simulink model "adc_to_xaui_v2_ddc"  (Simulink 6.2)
settings: Solver=ode45  StartTime=0.0  StopTime=100  RelTol=1e-3
undefined symbols (not defined in the file): BitWidth, iBOB
libraries: xbsIndex_r3 x168, casper_library x18, xps_library x5
(part 1 of 3)
settings Model: LastModifiedBy=siemion
settings DebuggingCC: SolverPrmCheckMsg=warning

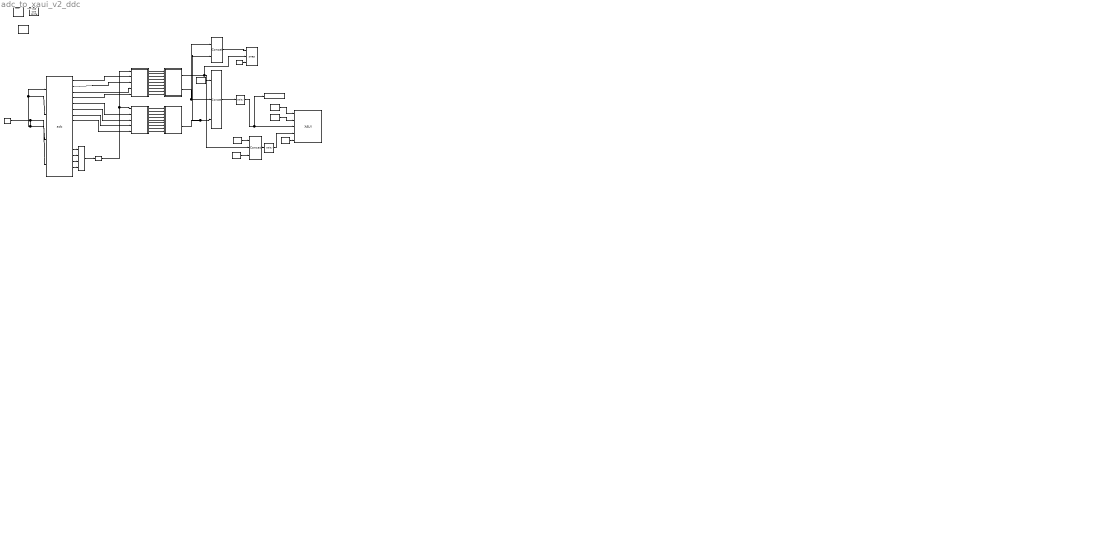
== system adc_to_xaui_v2_ddc ==
  note: left
  note: ADC-to-XAUI
      | Author: Peter McMahon
      | Version: 1.0
      | February 2008
  note: Beamformer Output:
      |
      | outofband[0]: 100PPS
      | outofband[1]: 1PPS
      | outofband[2-7]: unused
      |
      | data[0-7]: Pol 1 I
      | data[8-15]: Pol 1 Q
      | data[16-23]: Pol 2 I
      | data[24-31]: Pol 2 Q
      | data[31-63]: unused
  note: Used as a test device to emulate ATA beamformer.
      |
      | Digitizes data from 2x I/Q streams, and outputs them over XAUI.
  note: Pol 1
  note: Delay:
      | 1.) You always need at least one delay.
      | 2.) We want a delay of 5 to see if we can measure the
      | delay in the 1PPS in the ata_xaui design.
  " System Generator" : xbsIndex_r3/ System Generator  Tag=genX  xilinxfamily=Virtex2P  part=xc2vp50  speed=-7  package=ff1152  synthesis_tool=XST  directory=./adc_to_xaui_v2_ddc/sysgen  testbench=off  simulink_period=1  sysclk_period=8  incr_netlist=off  trim_vbits=Everywhere in SubSystem  dbl_ovrd=According to Block Masks  core_generation=According to Block Masks  run_coregen=off  deprecated_control=off  eval_field=0
      settings: AttributesFormatString=System\nGenerator
  Delay : xbsIndex_r3/Delay  latency=5  reg_retiming=off  explicit_period=off  period=1  en=off  accept_only_valid=off  init_zero=on  dbl_ovrd=off  show_param=off
      settings: xl_area=[0, 0, 0, 0, 0, 0, 0]
  Delay1 : xbsIndex_r3/Delay  latency=5  reg_retiming=off  explicit_period=off  period=1  en=off  accept_only_valid=off  init_zero=on  dbl_ovrd=off  show_param=off
      settings: xl_area=[0, 0, 0, 0, 0, 0, 0]
  XAUI : xps_library/XAUI  Tag=xps:xaui  demux=1  port=iBOB:1  show_param=on  pre_emph=2  swing=800
  XSG core config : xps_library/XSG core config  Tag=xps:xsg  hw_sys=iBOB  ibob_linux=off  clk_src=adc0_clk  gpio_clk_io_group=iBOB:sma  gpio_clk_bit_index=0  clk_rate=125  sample_period=1  synthesis_tool=XST  mpc_type=powerpc405
  adc : xps_library/adc  Tag=xps:adc  adc_brd=iBOB:adc0  adc_clk_rate=500  adc_interleave=off  sample_period=1
  cns0_2 : xbsIndex_r3/Constant  const=0  equ=P=C  arith_type=Boolean  n_bits=1  bin_pt=0  opselect=C  inp2=PCIN>>17  opr=+  inp1=P  carry=CIN  iostate=0  explicit_period=on  period=1  dbl_ovrd=off
  cns_xaui_data_32bits : xbsIndex_r3/Constant  const=0  equ=P=C  arith_type=Unsigned  n_bits=32  bin_pt=0  opselect=C  inp2=PCIN>>17  opr=+  inp1=P  carry=CIN  iostate=0  explicit_period=on  period=1  dbl_ovrd=off
  cns_xaui_outofband_1bit : xbsIndex_r3/Constant  const=0  equ=P=C  arith_type=Unsigned  n_bits=1  bin_pt=0  opselect=C  inp2=PCIN>>17  opr=+  inp1=P  carry=CIN  iostate=0  explicit_period=on  period=1  dbl_ovrd=off
  cns_xaui_outofband_6bits : xbsIndex_r3/Constant  const=0  equ=P=C  arith_type=Unsigned  n_bits=6  bin_pt=0  opselect=C  inp2=PCIN>>17  opr=+  inp1=P  carry=CIN  iostate=0  explicit_period=on  period=1  dbl_ovrd=off
  cns_xaui_rx_get : xbsIndex_r3/Constant  const=1  equ=P=C  arith_type=Boolean  n_bits=1  bin_pt=0  opselect=C  inp2=PCIN>>17  opr=+  inp1=P  carry=CIN  iostate=0  explicit_period=on  period=1  dbl_ovrd=off
  cns_xaui_rx_reset : xbsIndex_r3/Constant  const=0  equ=P=C  arith_type=Boolean  n_bits=1  bin_pt=0  opselect=C  inp2=PCIN>>17  opr=+  inp1=P  carry=CIN  iostate=0  explicit_period=on  period=1  dbl_ovrd=off
  cns_xaui_tx_valid : xbsIndex_r3/Constant  const=1  equ=P=C  arith_type=Boolean  n_bits=8  bin_pt=0  opselect=C  inp2=PCIN>>17  opr=+  inp1=P  carry=CIN  iostate=0  explicit_period=on  period=1  dbl_ovrd=off
  concat_data : xbsIndex_r3/Concat  num_inputs=3  explicit_period=off  period=1  dbl_ovrd=off
  concat_data1 : xbsIndex_r3/Concat  num_inputs=2  explicit_period=off  period=1  dbl_ovrd=off
  concat_outofband : xbsIndex_r3/Concat  num_inputs=3  explicit_period=off  period=1  dbl_ovrd=off
  dec_fir : Subsystem  AncestorBlock=casper_library/Downconverter/dec_fir  mask(dec_fir){n_inputs=4, coeff=.9 * [-0.0161   -0.0428   -0.0504   -0.0249    0.0354    0.1170    0.1948    0.2422    0.2422    0.1948    0.1170  0.0354   -0.0249   -0.0504   -0.0428   -0.0161], n_bits=8, quantization=Round  (unbiased: Even Values), add_latency=2, mult_latency=2}
      mask prompts: n_inputs "Number of Parallel Streams"; coeff "Coefficients"; n_bits "Bit Width Out"; quantization "Quantization Behavior"; add_latency "Add Latency"; mult_latency "Mult Latency"
      mask help: FIR filter which can handle multiple time samples in parallel and decimates down to 1 time sample. If coefficients are symmetric, will automatically fold before multiplying.
      mask init:
      | dec_fir_init(gcb, ...
      |     'n_inputs', n_inputs, ...
      |     'coeff', coeff, ...
      |     'n_bits', n_bits, ...
      |     'quantization', quantization, ...
      |     'add_latency', add_latency, ...
      |     'mult_latency', mult_latency);
      settings: AttributesFormatString=|
      | 16 taps
      | 8_7 r/i
      mask Help:
      | <h1>Description</h1>
      | 
      | FIR filter which can handle multiple time samples in parallel and decimates down to 1 time sample.  If coefficients are symmetric, will automatically fold before multiplying.
      | 
      | <h2>Mask Parameters</h2>
      | 
      | <b>Number of Parallel Streams</b> (n_inputs): The number of time samples which arrive in parallel.<br><br>
      | 
      | <b>Coefficients</b> (coeff): The FIR coefficients.  If this vector is symmetric, the FIR will automatically fold before multiplying.<br><br>
      | 
      | <b>Bit Width Out</b> (n_bits): The number of bits in each real/imag sample of the complex number that is output.<br><br>
      | 
      | <b>Quantization Behavior</b> (quantization): The quantization behavior used in converting to the output bit width.<br><br>
      | 
      | 
      | <b>Add Latency</b> (add_latency) = The latency of adders/converters.<br><br>
      | 
      | <b>Mult Latency</b> (mult_latency) = The latency of multipliers.<br><br>
      mask StyleString: edit,edit,edit,popup(Truncate|Round  (unbiased: +/- Inf)|Round  (unbiased: Even Values)),edit,edit
  dec_fir1 : Subsystem  AncestorBlock=casper_library/Downconverter/dec_fir  mask(dec_fir){n_inputs=4, coeff=.9 * [-0.0161   -0.0428   -0.0504   -0.0249    0.0354    0.1170    0.1948    0.2422    0.2422    0.1948    0.1170  0.0354   -0.0249   -0.0504   -0.0428   -0.0161], n_bits=8, quantization=Round  (unbiased: Even Values), add_latency=2, mult_latency=2}
      mask prompts: n_inputs "Number of Parallel Streams"; coeff "Coefficients"; n_bits "Bit Width Out"; quantization "Quantization Behavior"; add_latency "Add Latency"; mult_latency "Mult Latency"
      mask help: FIR filter which can handle multiple time samples in parallel and decimates down to 1 time sample. If coefficients are symmetric, will automatically fold before multiplying.
      mask init: same as adc_to_xaui_v2_ddc/dec_fir
      settings: AttributesFormatString=|
      | 16 taps
      | 8_7 r/i
      mask Help:
      | <h1>Description</h1>
      | 
      | FIR filter which can handle multiple time samples in parallel and decimates down to 1 time sample.  If coefficients are symmetric, will automatically fold before multiplying.
      | 
      | <h2>Mask Parameters</h2>
      | 
      | <b>Number of Parallel Streams</b> (n_inputs): The number of time samples which arrive in parallel.<br><br>
      | 
      | <b>Coefficients</b> (coeff): The FIR coefficients.  If this vector is symmetric, the FIR will automatically fold before multiplying.<br><br>
      | 
      | <b>Bit Width Out</b> (n_bits): The number of bits in each real/imag sample of the complex number that is output.<br><br>
      | 
      | <b>Quantization Behavior</b> (quantization): The quantization behavior used in converting to the output bit width.<br><br>
      | 
      | 
      | <b>Add Latency</b> (add_latency) = The latency of adders/converters.<br><br>
      | 
      | <b>Mult Latency</b> (mult_latency) = The latency of multipliers.<br><br>
      mask StyleString: edit,edit,edit,popup(Truncate|Round  (unbiased: +/- Inf)|Round  (unbiased: Even Values)),edit,edit
  ibob_lwip : xps_library/ibob_lwip
  mixer : Subsystem  AncestorBlock=casper_library/Downconverter/mixer  mask(mixer){freq_div=4, freq=1, nstreams=4, n_bits=8, bram_latency=2, mult_latency=3}
      mask prompts: freq_div "Frequency Divisions (M)"; freq "Mixing Frequency (? / M*2pi)"; nstreams "Number of Parallel Streams"; n_bits "Bit Width"; bram_latency "BRAM Latency"; mult_latency "Mult Latency"
      mask help: Digitally mixes an input signal (which can be several samples in parallel) with an LO of the indicated frequency (which is some fraction of the native FPGA clock rate).
      mask init:
      | mixer_init(gcb, ...
      |     'freq_div', freq_div, ...
      |     'freq', freq, ...
      |     'nstreams', nstreams, ...
      |     'n_bits', n_bits, ...
      |     'bram_latency', bram_latency, ...
      |     'mult_latency', mult_latency);
      settings: AttributesFormatString=lo at -1/4
      mask Help:
      | <h1>Description</h1>
      | 
      | Digitally mixes an input signal (which can be several samples in parallel) with an LO of the indicated frequency (which is some fraction of the native FPGA clock rate).
      | 
      | <h2>Mask Parameters</h2>
      | 
      | <b>Frequency Divisions</b> (freq_div):  The (power of 2) denominator of the mixing frequency. <br><br>
      | 
      | <b>Mixing Frequency</b> (freq) = The numerator of the mixing frequency.<br><br>
      | 
      | <b>Number of Parallel Streams</b> (nstreams) = The number of samples which arrive in parallel.<br><br>
      | 
      | <b>Bit Width</b> (n_bits) = The bitwidth of LO samples.<br><br>
      | 
      | <b>BRAM Latency</b> (bram_latency) = The latency of sine/cos lookup table.<br><br>
      | 
      | <b>MULT Latency</b> (mult_latency) = The latency of mixing multipliers.<br><br>
      | 
      | <h2> Usage </h2>
      | M = Frequency Divisions<br>
      | F = Mixing Frequency<br>
      | M and F must both be integers, and M must be a power of 2. The ratio F/M should equal the ratio f/r where r is the data rate of the sampled signal. For example, an F/M of 3/16 would downmix an 800Msps signal with an LO of 150MHz.
  mixer1 : Subsystem  AncestorBlock=casper_library/Downconverter/mixer  mask(mixer){freq_div=4, freq=1, nstreams=4, n_bits=8, bram_latency=2, mult_latency=3}
      mask prompts: freq_div "Frequency Divisions (M)"; freq "Mixing Frequency (? / M*2pi)"; nstreams "Number of Parallel Streams"; n_bits "Bit Width"; bram_latency "BRAM Latency"; mult_latency "Mult Latency"
      mask help: Digitally mixes an input signal (which can be several samples in parallel) with an LO of the indicated frequency (which is some fraction of the native FPGA clock rate).
      mask init: same as adc_to_xaui_v2_ddc/mixer
      settings: AttributesFormatString=lo at -1/4
      mask Help:
      | <h1>Description</h1>
      | 
      | Digitally mixes an input signal (which can be several samples in parallel) with an LO of the indicated frequency (which is some fraction of the native FPGA clock rate).
      | 
      | <h2>Mask Parameters</h2>
      | 
      | <b>Frequency Divisions</b> (freq_div):  The (power of 2) denominator of the mixing frequency. <br><br>
      | 
      | <b>Mixing Frequency</b> (freq) = The numerator of the mixing frequency.<br><br>
      | 
      | <b>Number of Parallel Streams</b> (nstreams) = The number of samples which arrive in parallel.<br><br>
      | 
      | <b>Bit Width</b> (n_bits) = The bitwidth of LO samples.<br><br>
      | 
      | <b>BRAM Latency</b> (bram_latency) = The latency of sine/cos lookup table.<br><br>
      | 
      | <b>MULT Latency</b> (mult_latency) = The latency of mixing multipliers.<br><br>
      | 
      | <h2> Usage </h2>
      | M = Frequency Divisions<br>
      | F = Mixing Frequency<br>
      | M and F must both be integers, and M must be a power of 2. The ratio F/M should equal the ratio f/r where r is the data rate of the sampled signal. For example, an F/M of 3/16 would downmix an 800Msps signal with an LO of 150MHz.
  posedge : casper_library/Misc/posedge  Tag=Rising Edge Detector
  reg_xauiscope1 : xps_library/software register  Tag=xps:sw_reg  io_dir=To Processor  arith_type=Unsigned  bitwidth=32  bin_pt=0  sample_period=1  gw_name=adc_to_xaui_v2_ddc_reg_xauiscope1_user_data_in
  sim_zero : Constant  Value=0
  snap_ddc : casper_library/Scopes/snap  nsamples=11
  sync_or : xbsIndex_r3/Logical  logical_function=OR  inputs=4  precision=Full  arith_type=Unsigned  n_bits=8  bin_pt=2  align_bp=on  latency=1  explicit_period=off  period=1  en=off  dbl_ovrd=off  show_param=off
      settings: xl_area=[0, 0, 0, 0, 0, 0, 0]
  wires:
  sim_zero/1 -> adc/4, adc/3, adc/2, adc/1
  adc/13 -> sync_or/1
  adc/14 -> sync_or/2
  adc/15 -> sync_or/3
  adc/16 -> sync_or/4
  sync_or/1 -> posedge/1
  cns_xaui_rx_get/1 -> XAUI/1
  cns_xaui_rx_reset/1 -> XAUI/2
  concat_outofband/1 -> Delay1/1
  cns_xaui_tx_valid/1 -> XAUI/5
  cns_xaui_data_32bits/1 -> concat_data/1
  cns_xaui_outofband_6bits/1 -> concat_outofband/1
  cns_xaui_outofband_1bit/1 -> concat_outofband/3
  concat_data/1 -> Delay/1
  Delay/1 -> XAUI/3, reg_xauiscope1/1
  Delay1/1 -> XAUI/4
  mixer/1(sync_out) -> dec_fir/1(sync_in)
  mixer/2(real1) -> dec_fir/2(real1)
  mixer/3(imag1) -> dec_fir/3(imag1)
  mixer/4(real2) -> dec_fir/4(real2)
  mixer/5(imag2) -> dec_fir/5(imag2)
  mixer/6(real3) -> dec_fir/6(real3)
  mixer/7(imag3) -> dec_fir/7(imag3)
  mixer/8(real4) -> dec_fir/8(real4)
  mixer/9(imag4) -> dec_fir/9(imag4)
  mixer1/1(sync_out) -> dec_fir1/1(sync_in)
  mixer1/2(real1) -> dec_fir1/2(real1)
  mixer1/3(imag1) -> dec_fir1/3(imag1)
  mixer1/4(real2) -> dec_fir1/4(real2)
  mixer1/5(imag2) -> dec_fir1/5(imag2)
  mixer1/6(real3) -> dec_fir1/6(real3)
  mixer1/7(imag3) -> dec_fir1/7(imag3)
  mixer1/8(real4) -> dec_fir1/8(real4)
  mixer1/9(imag4) -> dec_fir1/9(imag4)
  adc/1 -> mixer/2(din1)
  adc/2 -> mixer/3(din2)
  adc/3 -> mixer/4(din3)
  adc/4 -> mixer/5(din4)
  adc/5 -> mixer1/2(din1)
  adc/6 -> mixer1/3(din2)
  adc/7 -> mixer1/4(din3)
  adc/8 -> mixer1/5(din4)
  dec_fir/2(dout) -> concat_data/2, concat_data1/1
  dec_fir1/2(dout) -> concat_data/3, concat_data1/2
  posedge/1 -> mixer/1(sync), mixer1/1(sync)
  dec_fir/1(sync_out) -> concat_outofband/2, snap_ddc/2
  cns0_2/1 -> snap_ddc/3
  concat_data1/1 -> snap_ddc/1

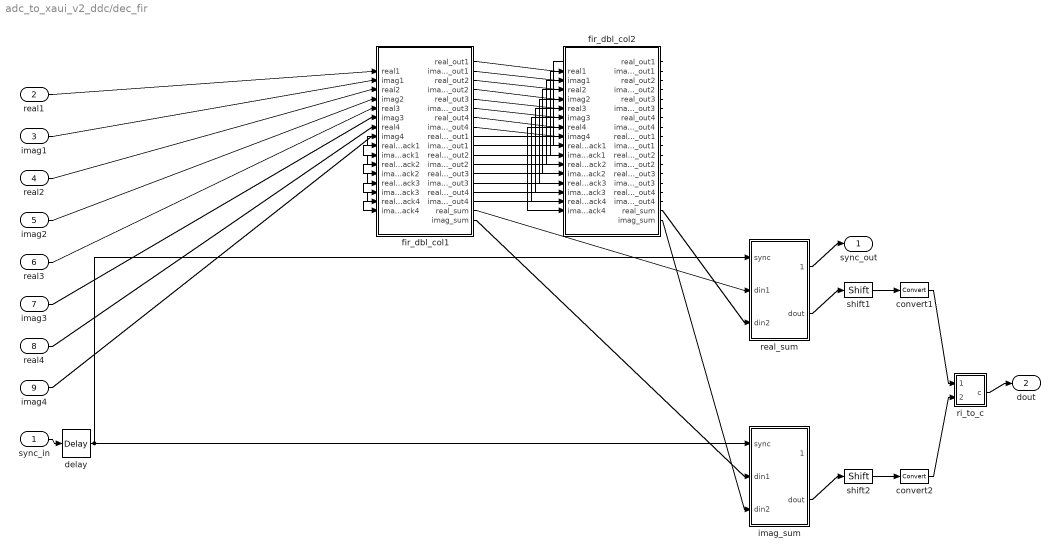
== system adc_to_xaui_v2_ddc/dec_fir ==
  sync_in : Inport  Port=1  LatchInput=off
  real1 : Inport  Port=2  LatchInput=off
  imag1 : Inport  Port=3  LatchInput=off
  real2 : Inport  Port=4  LatchInput=off
  imag2 : Inport  Port=5  LatchInput=off
  real3 : Inport  Port=6  LatchInput=off
  imag3 : Inport  Port=7  LatchInput=off
  real4 : Inport  Port=8  LatchInput=off
  imag4 : Inport  Port=9  LatchInput=off
  convert1 : xbsIndex_r3/Convert  arith_type="Signed  (2's comp)"  n_bits=8  bin_pt=7  quantization="Round  (unbiased: Even Values)"  overflow=Saturate  latency=2  explicit_period=on  period=1  dbl_ovrd=off  show_param=on  inserted_by_tool=off  pipeline=on
      settings: xl_area=[0, 0, 0, 0, 0, 0, 0]
  convert2 : xbsIndex_r3/Convert  arith_type="Signed  (2's comp)"  n_bits=8  bin_pt=7  quantization="Round  (unbiased: Even Values)"  overflow=Saturate  latency=2  explicit_period=on  period=1  dbl_ovrd=off  show_param=on  inserted_by_tool=off  pipeline=on
      settings: xl_area=[0, 0, 0, 0, 0, 0, 0]
  delay : xbsIndex_r3/Delay  latency=12  reg_retiming=off  explicit_period=off  period=1  en=off  accept_only_valid=off  init_zero=on  dbl_ovrd=off  show_param=off
      settings: xl_area=[0, 0, 0, 0, 0, 0, 0]
  fir_dbl_col1 : Subsystem  AncestorBlock=casper_library/Downconverter/fir_dbl_col  mask(fir_dbl_col){n_inputs=4, coeff=[-0.02241 -0.04536 -0.03852 -0.01449], add_latency=2, mult_latency=2}
      mask prompts: n_inputs "Inputs"; coeff "Coefficients"; add_latency "Add latency"; mult_latency "Mult Latency"
      mask init:
      | fir_dbl_col_init(gcb, ...
      |     'n_inputs', n_inputs, ...
      |     'coeff', coeff, ...
      |     'mult_latency', mult_latency, ...
      |     'add_latency', add_latency);
  fir_dbl_col2 : Subsystem  AncestorBlock=casper_library/Downconverter/fir_dbl_col  mask(fir_dbl_col){n_inputs=4, coeff=[0.21798 0.17532 0.1053 0.03186], add_latency=2, mult_latency=2}
      mask prompts: n_inputs "Inputs"; coeff "Coefficients"; add_latency "Add latency"; mult_latency "Mult Latency"
      mask init:
      | fir_dbl_col_init(gcb, ...
      |     'n_inputs', n_inputs, ...
      |     'coeff', coeff, ...
      |     'mult_latency', mult_latency, ...
      |     'add_latency', add_latency);
  imag_sum : Subsystem  AncestorBlock=casper_library/Misc/adder_tree  mask(adder_tree){n_inputs=2, latency=2}
      mask prompts: n_inputs "Number of Inputs"; latency "Add Latency"
      mask help: Sums all inputs using a tree of adds and delays.
      mask init:
      | adder_tree_init(gcb, ...
      |     'n_inputs', n_inputs, ...
      |     'latency', latency);
      settings: AttributesFormatString=latency 2
      mask Help: eval('xlWeb([getenv(''MLIB_ROOT''), ''\doc\html\sp_adder_tree\sp_adder_tree.html''])')
  real_sum : Subsystem  AncestorBlock=casper_library/Misc/adder_tree  mask(adder_tree){n_inputs=2, latency=2}
      mask prompts: n_inputs "Number of Inputs"; latency "Add Latency"
      mask help: Sums all inputs using a tree of adds and delays.
      mask init:
      | adder_tree_init(gcb, ...
      |     'n_inputs', n_inputs, ...
      |     'latency', latency);
      settings: AttributesFormatString=latency 2
      mask Help: eval('xlWeb([getenv(''MLIB_ROOT''), ''\doc\html\sp_adder_tree\sp_adder_tree.html''])')
  ri_to_c : Subsystem
  shift1 : xbsIndex_r3/Shift  shift_dir=Left  shift_bits=1  precision=Full  arith_type="Signed  (2's comp)"  n_bits=8  bin_pt=2  quantization=Truncate  overflow=Wrap  latency=0  explicit_period=off  period=1  en=off  dbl_ovrd=off  show_param=off
      settings: xl_area=[0, 0, 0, 0, 0, 0, 0]
  shift2 : xbsIndex_r3/Shift  shift_dir=Left  shift_bits=1  precision=Full  arith_type="Signed  (2's comp)"  n_bits=8  bin_pt=2  quantization=Truncate  overflow=Wrap  latency=0  explicit_period=off  period=1  en=off  dbl_ovrd=off  show_param=off
      settings: xl_area=[0, 0, 0, 0, 0, 0, 0]
  sync_out : Outport
  dout : Outport  Port=2
  wires:
  real1/1 -> fir_dbl_col1/1(real1)
  imag1/1 -> fir_dbl_col1/2(imag1)
  real2/1 -> fir_dbl_col1/3(real2)
  imag2/1 -> fir_dbl_col1/4(imag2)
  real3/1 -> fir_dbl_col1/5(real3)
  imag3/1 -> fir_dbl_col1/6(imag3)
  real4/1 -> fir_dbl_col1/7(real4)
  imag4/1 -> fir_dbl_col1/8(imag4)
  fir_dbl_col1/17(real_sum) -> real_sum/2(din1)
  fir_dbl_col1/18(imag_sum) -> imag_sum/2(din1)
  fir_dbl_col1/1(real_out1) -> fir_dbl_col2/1(real1)
  fir_dbl_col1/2(imag_out1) -> fir_dbl_col2/2(imag1)
  fir_dbl_col1/3(real_out2) -> fir_dbl_col2/3(real2)
  fir_dbl_col1/4(imag_out2) -> fir_dbl_col2/4(imag2)
  fir_dbl_col1/5(real_out3) -> fir_dbl_col2/5(real3)
  fir_dbl_col1/6(imag_out3) -> fir_dbl_col2/6(imag3)
  fir_dbl_col1/7(real_out4) -> fir_dbl_col2/7(real4)
  fir_dbl_col1/8(imag_out4) -> fir_dbl_col2/8(imag4)
  fir_dbl_col2/17(real_sum) -> real_sum/3(din2)
  fir_dbl_col2/18(imag_sum) -> imag_sum/3(din2)
  real_sum/2(dout) -> shift1/1
  imag_sum/2(dout) -> shift2/1
  shift1/1 -> convert1/1
  shift2/1 -> convert2/1
  convert1/1 -> ri_to_c/1(re)
  convert2/1 -> ri_to_c/2(im)
  ri_to_c/1(c) -> dout/1
  sync_in/1 -> delay/1
  delay/1 -> real_sum/1(sync), imag_sum/1(sync)
  real_sum/1(sync_out) -> sync_out/1
  fir_dbl_col2/9(real_back_out1) -> fir_dbl_col1/9(real_back1)
  fir_dbl_col2/10(imag_back_out1) -> fir_dbl_col1/10(imag_back1)
  fir_dbl_col2/11(real_back_out2) -> fir_dbl_col1/11(real_back2)
  fir_dbl_col2/12(imag_back_out2) -> fir_dbl_col1/12(imag_back2)
  fir_dbl_col2/13(real_back_out3) -> fir_dbl_col1/13(real_back3)
  fir_dbl_col2/14(imag_back_out3) -> fir_dbl_col1/14(imag_back3)
  fir_dbl_col2/15(real_back_out4) -> fir_dbl_col1/15(real_back4)
  fir_dbl_col2/16(imag_back_out4) -> fir_dbl_col1/16(imag_back4)
  fir_dbl_col2/1(real_out1) -> fir_dbl_col2/9(real_back1)
  fir_dbl_col2/2(imag_out1) -> fir_dbl_col2/10(imag_back1)
  fir_dbl_col2/3(real_out2) -> fir_dbl_col2/11(real_back2)
  fir_dbl_col2/4(imag_out2) -> fir_dbl_col2/12(imag_back2)
  fir_dbl_col2/5(real_out3) -> fir_dbl_col2/13(real_back3)
  fir_dbl_col2/6(imag_out3) -> fir_dbl_col2/14(imag_back3)
  fir_dbl_col2/7(real_out4) -> fir_dbl_col2/15(real_back4)
  fir_dbl_col2/8(imag_out4) -> fir_dbl_col2/16(imag_back4)

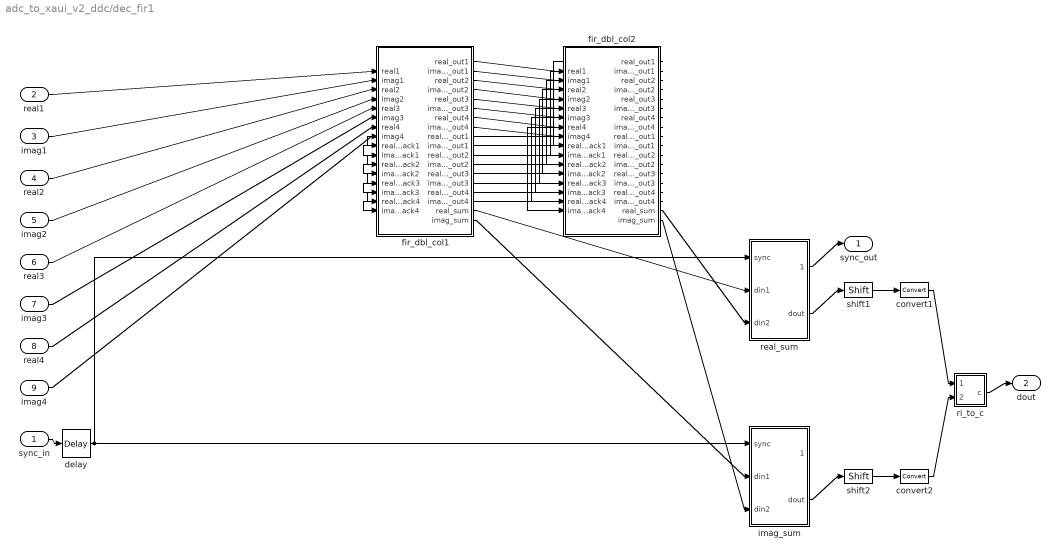
== system adc_to_xaui_v2_ddc/dec_fir1 ==
  sync_in : Inport  Port=1  LatchInput=off
  real1 : Inport  Port=2  LatchInput=off
  imag1 : Inport  Port=3  LatchInput=off
  real2 : Inport  Port=4  LatchInput=off
  imag2 : Inport  Port=5  LatchInput=off
  real3 : Inport  Port=6  LatchInput=off
  imag3 : Inport  Port=7  LatchInput=off
  real4 : Inport  Port=8  LatchInput=off
  imag4 : Inport  Port=9  LatchInput=off
  convert1 : xbsIndex_r3/Convert  arith_type="Signed  (2's comp)"  n_bits=8  bin_pt=7  quantization="Round  (unbiased: Even Values)"  overflow=Saturate  latency=2  explicit_period=on  period=1  dbl_ovrd=off  show_param=on  inserted_by_tool=off  pipeline=on
      settings: xl_area=[0, 0, 0, 0, 0, 0, 0]
  convert2 : xbsIndex_r3/Convert  arith_type="Signed  (2's comp)"  n_bits=8  bin_pt=7  quantization="Round  (unbiased: Even Values)"  overflow=Saturate  latency=2  explicit_period=on  period=1  dbl_ovrd=off  show_param=on  inserted_by_tool=off  pipeline=on
      settings: xl_area=[0, 0, 0, 0, 0, 0, 0]
  delay : xbsIndex_r3/Delay  latency=12  reg_retiming=off  explicit_period=off  period=1  en=off  accept_only_valid=off  init_zero=on  dbl_ovrd=off  show_param=off
      settings: xl_area=[0, 0, 0, 0, 0, 0, 0]
  fir_dbl_col1 : Subsystem  AncestorBlock=casper_library/Downconverter/fir_dbl_col  mask(fir_dbl_col){n_inputs=4, coeff=[-0.02241 -0.04536 -0.03852 -0.01449], add_latency=2, mult_latency=2}
      mask prompts: n_inputs "Inputs"; coeff "Coefficients"; add_latency "Add latency"; mult_latency "Mult Latency"
      mask init:
      | fir_dbl_col_init(gcb, ...
      |     'n_inputs', n_inputs, ...
      |     'coeff', coeff, ...
      |     'mult_latency', mult_latency, ...
      |     'add_latency', add_latency);
  fir_dbl_col2 : Subsystem  AncestorBlock=casper_library/Downconverter/fir_dbl_col  mask(fir_dbl_col){n_inputs=4, coeff=[0.21798 0.17532 0.1053 0.03186], add_latency=2, mult_latency=2}
      mask prompts: n_inputs "Inputs"; coeff "Coefficients"; add_latency "Add latency"; mult_latency "Mult Latency"
      mask init:
      | fir_dbl_col_init(gcb, ...
      |     'n_inputs', n_inputs, ...
      |     'coeff', coeff, ...
      |     'mult_latency', mult_latency, ...
      |     'add_latency', add_latency);
  imag_sum : Subsystem  AncestorBlock=casper_library/Misc/adder_tree  mask(adder_tree){n_inputs=2, latency=2}
      mask prompts: n_inputs "Number of Inputs"; latency "Add Latency"
      mask help: Sums all inputs using a tree of adds and delays.
      mask init:
      | adder_tree_init(gcb, ...
      |     'n_inputs', n_inputs, ...
      |     'latency', latency);
      settings: AttributesFormatString=latency 2
      mask Help: eval('xlWeb([getenv(''MLIB_ROOT''), ''\doc\html\sp_adder_tree\sp_adder_tree.html''])')
  real_sum : Subsystem  AncestorBlock=casper_library/Misc/adder_tree  mask(adder_tree){n_inputs=2, latency=2}
      mask prompts: n_inputs "Number of Inputs"; latency "Add Latency"
      mask help: Sums all inputs using a tree of adds and delays.
      mask init:
      | adder_tree_init(gcb, ...
      |     'n_inputs', n_inputs, ...
      |     'latency', latency);
      settings: AttributesFormatString=latency 2
      mask Help: eval('xlWeb([getenv(''MLIB_ROOT''), ''\doc\html\sp_adder_tree\sp_adder_tree.html''])')
  ri_to_c : Subsystem
  shift1 : xbsIndex_r3/Shift  shift_dir=Left  shift_bits=1  precision=Full  arith_type="Signed  (2's comp)"  n_bits=8  bin_pt=2  quantization=Truncate  overflow=Wrap  latency=0  explicit_period=off  period=1  en=off  dbl_ovrd=off  show_param=off
      settings: xl_area=[0, 0, 0, 0, 0, 0, 0]
  shift2 : xbsIndex_r3/Shift  shift_dir=Left  shift_bits=1  precision=Full  arith_type="Signed  (2's comp)"  n_bits=8  bin_pt=2  quantization=Truncate  overflow=Wrap  latency=0  explicit_period=off  period=1  en=off  dbl_ovrd=off  show_param=off
      settings: xl_area=[0, 0, 0, 0, 0, 0, 0]
  sync_out : Outport
  dout : Outport  Port=2
  wires:
  real1/1 -> fir_dbl_col1/1(real1)
  imag1/1 -> fir_dbl_col1/2(imag1)
  real2/1 -> fir_dbl_col1/3(real2)
  imag2/1 -> fir_dbl_col1/4(imag2)
  real3/1 -> fir_dbl_col1/5(real3)
  imag3/1 -> fir_dbl_col1/6(imag3)
  real4/1 -> fir_dbl_col1/7(real4)
  imag4/1 -> fir_dbl_col1/8(imag4)
  fir_dbl_col1/17(real_sum) -> real_sum/2(din1)
  fir_dbl_col1/18(imag_sum) -> imag_sum/2(din1)
  fir_dbl_col1/1(real_out1) -> fir_dbl_col2/1(real1)
  fir_dbl_col1/2(imag_out1) -> fir_dbl_col2/2(imag1)
  fir_dbl_col1/3(real_out2) -> fir_dbl_col2/3(real2)
  fir_dbl_col1/4(imag_out2) -> fir_dbl_col2/4(imag2)
  fir_dbl_col1/5(real_out3) -> fir_dbl_col2/5(real3)
  fir_dbl_col1/6(imag_out3) -> fir_dbl_col2/6(imag3)
  fir_dbl_col1/7(real_out4) -> fir_dbl_col2/7(real4)
  fir_dbl_col1/8(imag_out4) -> fir_dbl_col2/8(imag4)
  fir_dbl_col2/17(real_sum) -> real_sum/3(din2)
  fir_dbl_col2/18(imag_sum) -> imag_sum/3(din2)
  real_sum/2(dout) -> shift1/1
  imag_sum/2(dout) -> shift2/1
  shift1/1 -> convert1/1
  shift2/1 -> convert2/1
  convert1/1 -> ri_to_c/1(re)
  convert2/1 -> ri_to_c/2(im)
  ri_to_c/1(c) -> dout/1
  sync_in/1 -> delay/1
  delay/1 -> real_sum/1(sync), imag_sum/1(sync)
  real_sum/1(sync_out) -> sync_out/1
  fir_dbl_col2/9(real_back_out1) -> fir_dbl_col1/9(real_back1)
  fir_dbl_col2/10(imag_back_out1) -> fir_dbl_col1/10(imag_back1)
  fir_dbl_col2/11(real_back_out2) -> fir_dbl_col1/11(real_back2)
  fir_dbl_col2/12(imag_back_out2) -> fir_dbl_col1/12(imag_back2)
  fir_dbl_col2/13(real_back_out3) -> fir_dbl_col1/13(real_back3)
  fir_dbl_col2/14(imag_back_out3) -> fir_dbl_col1/14(imag_back3)
  fir_dbl_col2/15(real_back_out4) -> fir_dbl_col1/15(real_back4)
  fir_dbl_col2/16(imag_back_out4) -> fir_dbl_col1/16(imag_back4)
  fir_dbl_col2/1(real_out1) -> fir_dbl_col2/9(real_back1)
  fir_dbl_col2/2(imag_out1) -> fir_dbl_col2/10(imag_back1)
  fir_dbl_col2/3(real_out2) -> fir_dbl_col2/11(real_back2)
  fir_dbl_col2/4(imag_out2) -> fir_dbl_col2/12(imag_back2)
  fir_dbl_col2/5(real_out3) -> fir_dbl_col2/13(real_back3)
  fir_dbl_col2/6(imag_out3) -> fir_dbl_col2/14(imag_back3)
  fir_dbl_col2/7(real_out4) -> fir_dbl_col2/15(real_back4)
  fir_dbl_col2/8(imag_out4) -> fir_dbl_col2/16(imag_back4)

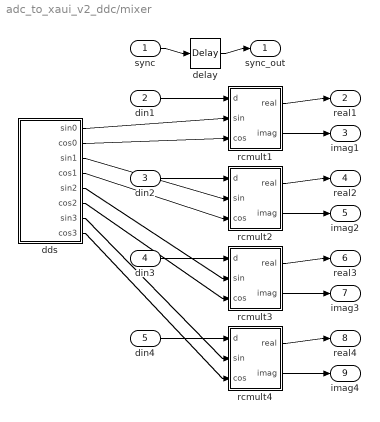
== system adc_to_xaui_v2_ddc/mixer ==
  sync : Inport  Port=1  LatchInput=off
  din1 : Inport  Port=2  LatchInput=off
  din2 : Inport  Port=3  LatchInput=off
  din3 : Inport  Port=4  LatchInput=off
  din4 : Inport  Port=5  LatchInput=off
  dds : Subsystem  AncestorBlock=casper_library/Downconverter/dds  mask(dds){freq_div=4, freq=1, num_lo=4, n_bits=8, latency=2}
      mask prompts: freq_div "Frequency divisions (M)"; freq "Frequency (? / M*2pi)"; num_lo "Parallel LOs"; n_bits "Bit Width"
      mask init:
      | dds_init(gcb, ...
      |     'freq_div', freq_div, ...
      |     'freq', freq, ...
      |     'num_lo', num_lo, ...
      |     'n_bits', n_bits, ...
      |     'latency', latency);
      settings: AttributesFormatString=lo at -1/4
  delay : xbsIndex_r3/Delay  latency=3  reg_retiming=off  explicit_period=off  period=1  en=off  accept_only_valid=off  init_zero=on  dbl_ovrd=off  show_param=off
      settings: xl_area=[0, 0, 0, 0, 0, 0, 0]
  rcmult1 : Subsystem  AncestorBlock=casper_library/Downconverter/rcmult  mask(rcmult){latency=3}
  rcmult2 : Subsystem  AncestorBlock=casper_library/Downconverter/rcmult  mask(rcmult){latency=3}
  rcmult3 : Subsystem  AncestorBlock=casper_library/Downconverter/rcmult  mask(rcmult){latency=3}
  rcmult4 : Subsystem  AncestorBlock=casper_library/Downconverter/rcmult  mask(rcmult){latency=3}
  sync_out : Outport
  real1 : Outport  Port=2
  imag1 : Outport  Port=3
  real2 : Outport  Port=4
  imag2 : Outport  Port=5
  real3 : Outport  Port=6
  imag3 : Outport  Port=7
  real4 : Outport  Port=8
  imag4 : Outport  Port=9
  wires:
  sync/1 -> delay/1
  delay/1 -> sync_out/1
  din1/1 -> rcmult1/1(d)
  dds/1(sin0) -> rcmult1/2(sin)
  dds/2(cos0) -> rcmult1/3(cos)
  rcmult1/1(real) -> real1/1
  rcmult1/2(imag) -> imag1/1
  din2/1 -> rcmult2/1(d)
  dds/3(sin1) -> rcmult2/2(sin)
  dds/4(cos1) -> rcmult2/3(cos)
  rcmult2/1(real) -> real2/1
  rcmult2/2(imag) -> imag2/1
  din3/1 -> rcmult3/1(d)
  dds/5(sin2) -> rcmult3/2(sin)
  dds/6(cos2) -> rcmult3/3(cos)
  rcmult3/1(real) -> real3/1
  rcmult3/2(imag) -> imag3/1
  din4/1 -> rcmult4/1(d)
  dds/7(sin3) -> rcmult4/2(sin)
  dds/8(cos3) -> rcmult4/3(cos)
  rcmult4/1(real) -> real4/1
  rcmult4/2(imag) -> imag4/1

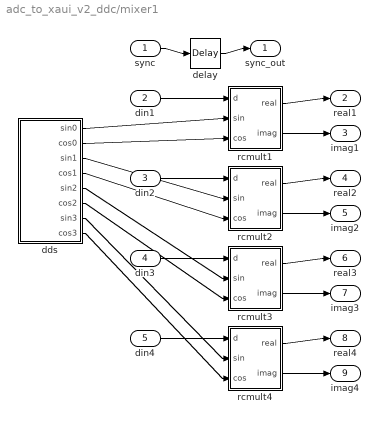
== system adc_to_xaui_v2_ddc/mixer1 ==
  sync : Inport  Port=1  LatchInput=off
  din1 : Inport  Port=2  LatchInput=off
  din2 : Inport  Port=3  LatchInput=off
  din3 : Inport  Port=4  LatchInput=off
  din4 : Inport  Port=5  LatchInput=off
  dds : Subsystem  AncestorBlock=casper_library/Downconverter/dds  mask(dds){freq_div=4, freq=1, num_lo=4, n_bits=8, latency=2}
      mask prompts: freq_div "Frequency divisions (M)"; freq "Frequency (? / M*2pi)"; num_lo "Parallel LOs"; n_bits "Bit Width"
      mask init:
      | dds_init(gcb, ...
      |     'freq_div', freq_div, ...
      |     'freq', freq, ...
      |     'num_lo', num_lo, ...
      |     'n_bits', n_bits, ...
      |     'latency', latency);
      settings: AttributesFormatString=lo at -1/4
  delay : xbsIndex_r3/Delay  latency=3  reg_retiming=off  explicit_period=off  period=1  en=off  accept_only_valid=off  init_zero=on  dbl_ovrd=off  show_param=off
      settings: xl_area=[0, 0, 0, 0, 0, 0, 0]
  rcmult1 : Subsystem  AncestorBlock=casper_library/Downconverter/rcmult  mask(rcmult){latency=3}
  rcmult2 : Subsystem  AncestorBlock=casper_library/Downconverter/rcmult  mask(rcmult){latency=3}
  rcmult3 : Subsystem  AncestorBlock=casper_library/Downconverter/rcmult  mask(rcmult){latency=3}
  rcmult4 : Subsystem  AncestorBlock=casper_library/Downconverter/rcmult  mask(rcmult){latency=3}
  sync_out : Outport
  real1 : Outport  Port=2
  imag1 : Outport  Port=3
  real2 : Outport  Port=4
  imag2 : Outport  Port=5
  real3 : Outport  Port=6
  imag3 : Outport  Port=7
  real4 : Outport  Port=8
  imag4 : Outport  Port=9
  wires:
  sync/1 -> delay/1
  delay/1 -> sync_out/1
  din1/1 -> rcmult1/1(d)
  dds/1(sin0) -> rcmult1/2(sin)
  dds/2(cos0) -> rcmult1/3(cos)
  rcmult1/1(real) -> real1/1
  rcmult1/2(imag) -> imag1/1
  din2/1 -> rcmult2/1(d)
  dds/3(sin1) -> rcmult2/2(sin)
  dds/4(cos1) -> rcmult2/3(cos)
  rcmult2/1(real) -> real2/1
  rcmult2/2(imag) -> imag2/1
  din3/1 -> rcmult3/1(d)
  dds/5(sin2) -> rcmult3/2(sin)
  dds/6(cos2) -> rcmult3/3(cos)
  rcmult3/1(real) -> real3/1
  rcmult3/2(imag) -> imag3/1
  din4/1 -> rcmult4/1(d)
  dds/7(sin3) -> rcmult4/2(sin)
  dds/8(cos3) -> rcmult4/3(cos)
  rcmult4/1(real) -> real4/1
  rcmult4/2(imag) -> imag4/1

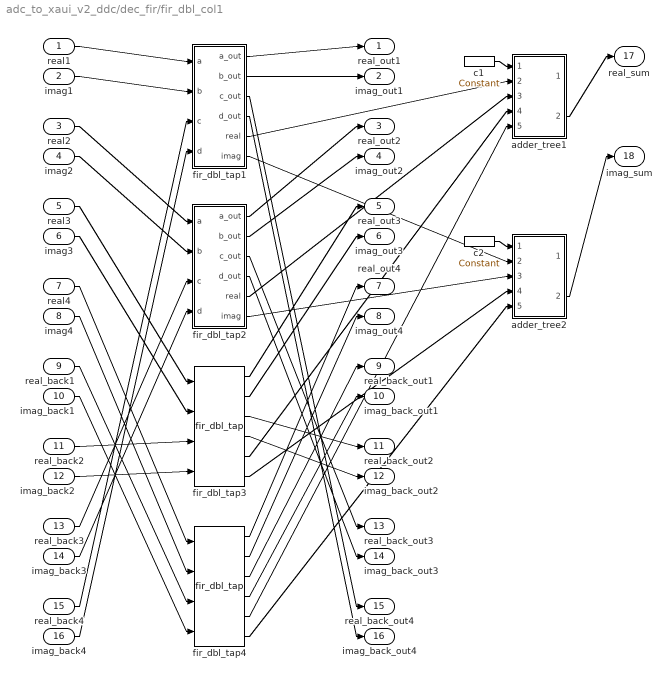
== system adc_to_xaui_v2_ddc/dec_fir/fir_dbl_col1 ==
  real1 : Inport  Port=1  LatchInput=off
  imag1 : Inport  Port=2  LatchInput=off
  real2 : Inport  Port=3  LatchInput=off
  imag2 : Inport  Port=4  LatchInput=off
  real3 : Inport  Port=5  LatchInput=off
  imag3 : Inport  Port=6  LatchInput=off
  real4 : Inport  Port=7  LatchInput=off
  imag4 : Inport  Port=8  LatchInput=off
  real_back1 : Inport  Port=9  LatchInput=off
  imag_back1 : Inport  Port=10  LatchInput=off
  real_back2 : Inport  Port=11  LatchInput=off
  imag_back2 : Inport  Port=12  LatchInput=off
  real_back3 : Inport  Port=13  LatchInput=off
  imag_back3 : Inport  Port=14  LatchInput=off
  real_back4 : Inport  Port=15  LatchInput=off
  imag_back4 : Inport  Port=16  LatchInput=off
  adder_tree1 : Subsystem  AncestorBlock=casper_library/Misc/adder_tree  mask(adder_tree){n_inputs=4, latency=2}
      mask prompts: n_inputs "Number of Inputs"; latency "Add Latency"
      mask help: Sums all inputs using a tree of adds and delays.
      mask init:
      | adder_tree_init(gcb, ...
      |     'n_inputs', n_inputs, ...
      |     'latency', latency);
      settings: AttributesFormatString=latency 4
      mask Help: eval('xlWeb([getenv(''MLIB_ROOT''), ''\doc\html\sp_adder_tree\sp_adder_tree.html''])')
  adder_tree2 : Subsystem  AncestorBlock=casper_library/Misc/adder_tree  mask(adder_tree){n_inputs=4, latency=2}
      mask prompts: n_inputs "Number of Inputs"; latency "Add Latency"
      mask help: Sums all inputs using a tree of adds and delays.
      mask init:
      | adder_tree_init(gcb, ...
      |     'n_inputs', n_inputs, ...
      |     'latency', latency);
      settings: AttributesFormatString=latency 4
      mask Help: eval('xlWeb([getenv(''MLIB_ROOT''), ''\doc\html\sp_adder_tree\sp_adder_tree.html''])')
  c1 : xbsIndex_r3/Constant  const=1  equ=P=C  arith_type=Unsigned  n_bits=1  bin_pt=0  opselect=C  inp2=PCIN>>17  opr=+  inp1=P  carry=CIN  iostate=0  explicit_period=on  period=1  dbl_ovrd=off
  c2 : xbsIndex_r3/Constant  const=1  equ=P=C  arith_type=Unsigned  n_bits=1  bin_pt=0  opselect=C  inp2=PCIN>>17  opr=+  inp1=P  carry=CIN  iostate=0  explicit_period=on  period=1  dbl_ovrd=off
  fir_dbl_tap1 : Subsystem  AncestorBlock=casper_library/Downconverter/fir_dbl_tap  mask(fir_dbl_tap){factor=-0.02241, add_latency=2, mult_latency=2}
      mask prompts: add_latency "Add latency"; mult_latency "Mult latency"
  fir_dbl_tap2 : Subsystem  AncestorBlock=casper_library/Downconverter/fir_dbl_tap  mask(fir_dbl_tap){factor=-0.04536, add_latency=2, mult_latency=2}
      mask prompts: add_latency "Add latency"; mult_latency "Mult latency"
  fir_dbl_tap3 : casper_library/Downconverter/fir_dbl_tap  factor=-0.03852  add_latency=2  mult_latency=2
      link override Constant: equ=P=C
  fir_dbl_tap4 : casper_library/Downconverter/fir_dbl_tap  factor=-0.01449  add_latency=2  mult_latency=2
      link override Constant: equ=P=C
  real_out1 : Outport
  imag_out1 : Outport  Port=2
  real_out2 : Outport  Port=3
  imag_out2 : Outport  Port=4
  real_out3 : Outport  Port=5
  imag_out3 : Outport  Port=6
  real_out4 : Outport  Port=7
  imag_out4 : Outport  Port=8
  real_back_out1 : Outport  Port=9
  imag_back_out1 : Outport  Port=10
  real_back_out2 : Outport  Port=11
  imag_back_out2 : Outport  Port=12
  real_back_out3 : Outport  Port=13
  imag_back_out3 : Outport  Port=14
  real_back_out4 : Outport  Port=15
  imag_back_out4 : Outport  Port=16
  real_sum : Outport  Port=17
  imag_sum : Outport  Port=18
  wires:
  c1/1 -> adder_tree1/1(sync)
  c2/1 -> adder_tree2/1(sync)
  adder_tree1/2(dout) -> real_sum/1
  adder_tree2/2(dout) -> imag_sum/1
  real1/1 -> fir_dbl_tap1/1(a)
  imag1/1 -> fir_dbl_tap1/2(b)
  real_back4/1 -> fir_dbl_tap1/3(c)
  imag_back4/1 -> fir_dbl_tap1/4(d)
  fir_dbl_tap1/1(a_out) -> real_out1/1
  fir_dbl_tap1/2(b_out) -> imag_out1/1
  fir_dbl_tap1/3(c_out) -> real_back_out4/1
  fir_dbl_tap1/4(d_out) -> imag_back_out4/1
  fir_dbl_tap1/5(real) -> adder_tree1/2(din1)
  fir_dbl_tap1/6(imag) -> adder_tree2/2(din1)
  real2/1 -> fir_dbl_tap2/1(a)
  imag2/1 -> fir_dbl_tap2/2(b)
  real_back3/1 -> fir_dbl_tap2/3(c)
  imag_back3/1 -> fir_dbl_tap2/4(d)
  fir_dbl_tap2/1(a_out) -> real_out2/1
  fir_dbl_tap2/2(b_out) -> imag_out2/1
  fir_dbl_tap2/3(c_out) -> real_back_out3/1
  fir_dbl_tap2/4(d_out) -> imag_back_out3/1
  fir_dbl_tap2/5(real) -> adder_tree1/3(din2)
  fir_dbl_tap2/6(imag) -> adder_tree2/3(din2)
  real3/1 -> fir_dbl_tap3/1
  imag3/1 -> fir_dbl_tap3/2
  real_back2/1 -> fir_dbl_tap3/3
  imag_back2/1 -> fir_dbl_tap3/4
  fir_dbl_tap3/1 -> real_out3/1
  fir_dbl_tap3/2 -> imag_out3/1
  fir_dbl_tap3/3 -> real_back_out2/1
  fir_dbl_tap3/4 -> imag_back_out2/1
  fir_dbl_tap3/5 -> adder_tree1/4(din3)
  fir_dbl_tap3/6 -> adder_tree2/4(din3)
  real4/1 -> fir_dbl_tap4/1
  imag4/1 -> fir_dbl_tap4/2
  real_back1/1 -> fir_dbl_tap4/3
  imag_back1/1 -> fir_dbl_tap4/4
  fir_dbl_tap4/1 -> real_out4/1
  fir_dbl_tap4/2 -> imag_out4/1
  fir_dbl_tap4/3 -> real_back_out1/1
  fir_dbl_tap4/4 -> imag_back_out1/1
  fir_dbl_tap4/5 -> adder_tree1/5(din4)
  fir_dbl_tap4/6 -> adder_tree2/5(din4)

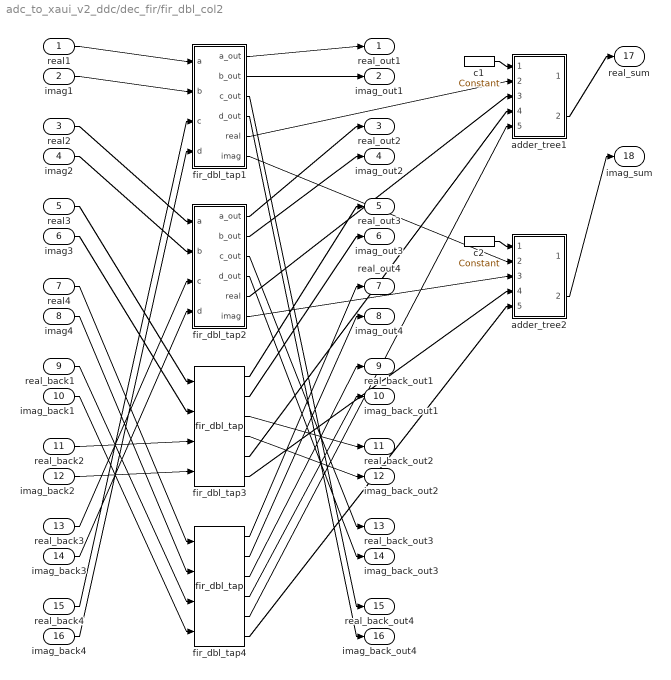
== system adc_to_xaui_v2_ddc/dec_fir/fir_dbl_col2 ==
  real1 : Inport  Port=1  LatchInput=off
  imag1 : Inport  Port=2  LatchInput=off
  real2 : Inport  Port=3  LatchInput=off
  imag2 : Inport  Port=4  LatchInput=off
  real3 : Inport  Port=5  LatchInput=off
  imag3 : Inport  Port=6  LatchInput=off
  real4 : Inport  Port=7  LatchInput=off
  imag4 : Inport  Port=8  LatchInput=off
  real_back1 : Inport  Port=9  LatchInput=off
  imag_back1 : Inport  Port=10  LatchInput=off
  real_back2 : Inport  Port=11  LatchInput=off
  imag_back2 : Inport  Port=12  LatchInput=off
  real_back3 : Inport  Port=13  LatchInput=off
  imag_back3 : Inport  Port=14  LatchInput=off
  real_back4 : Inport  Port=15  LatchInput=off
  imag_back4 : Inport  Port=16  LatchInput=off
  adder_tree1 : Subsystem  AncestorBlock=casper_library/Misc/adder_tree  mask(adder_tree){n_inputs=4, latency=2}
      mask prompts: n_inputs "Number of Inputs"; latency "Add Latency"
      mask help: Sums all inputs using a tree of adds and delays.
      mask init:
      | adder_tree_init(gcb, ...
      |     'n_inputs', n_inputs, ...
      |     'latency', latency);
      settings: AttributesFormatString=latency 4
      mask Help: eval('xlWeb([getenv(''MLIB_ROOT''), ''\doc\html\sp_adder_tree\sp_adder_tree.html''])')
  adder_tree2 : Subsystem  AncestorBlock=casper_library/Misc/adder_tree  mask(adder_tree){n_inputs=4, latency=2}
      mask prompts: n_inputs "Number of Inputs"; latency "Add Latency"
      mask help: Sums all inputs using a tree of adds and delays.
      mask init:
      | adder_tree_init(gcb, ...
      |     'n_inputs', n_inputs, ...
      |     'latency', latency);
      settings: AttributesFormatString=latency 4
      mask Help: eval('xlWeb([getenv(''MLIB_ROOT''), ''\doc\html\sp_adder_tree\sp_adder_tree.html''])')
  c1 : xbsIndex_r3/Constant  const=1  equ=P=C  arith_type=Unsigned  n_bits=1  bin_pt=0  opselect=C  inp2=PCIN>>17  opr=+  inp1=P  carry=CIN  iostate=0  explicit_period=on  period=1  dbl_ovrd=off
  c2 : xbsIndex_r3/Constant  const=1  equ=P=C  arith_type=Unsigned  n_bits=1  bin_pt=0  opselect=C  inp2=PCIN>>17  opr=+  inp1=P  carry=CIN  iostate=0  explicit_period=on  period=1  dbl_ovrd=off
  fir_dbl_tap1 : Subsystem  AncestorBlock=casper_library/Downconverter/fir_dbl_tap  mask(fir_dbl_tap){factor=0.21798, add_latency=2, mult_latency=2}
      mask prompts: add_latency "Add latency"; mult_latency "Mult latency"
  fir_dbl_tap2 : Subsystem  AncestorBlock=casper_library/Downconverter/fir_dbl_tap  mask(fir_dbl_tap){factor=0.17532, add_latency=2, mult_latency=2}
      mask prompts: add_latency "Add latency"; mult_latency "Mult latency"
  fir_dbl_tap3 : casper_library/Downconverter/fir_dbl_tap  factor=0.1053  add_latency=2  mult_latency=2
      link override Constant: equ=P=C
  fir_dbl_tap4 : casper_library/Downconverter/fir_dbl_tap  factor=0.03186  add_latency=2  mult_latency=2
      link override Constant: equ=P=C
  real_out1 : Outport
  imag_out1 : Outport  Port=2
  real_out2 : Outport  Port=3
  imag_out2 : Outport  Port=4
  real_out3 : Outport  Port=5
  imag_out3 : Outport  Port=6
  real_out4 : Outport  Port=7
  imag_out4 : Outport  Port=8
  real_back_out1 : Outport  Port=9
  imag_back_out1 : Outport  Port=10
  real_back_out2 : Outport  Port=11
  imag_back_out2 : Outport  Port=12
  real_back_out3 : Outport  Port=13
  imag_back_out3 : Outport  Port=14
  real_back_out4 : Outport  Port=15
  imag_back_out4 : Outport  Port=16
  real_sum : Outport  Port=17
  imag_sum : Outport  Port=18
  wires:
  c1/1 -> adder_tree1/1(sync)
  c2/1 -> adder_tree2/1(sync)
  adder_tree1/2(dout) -> real_sum/1
  adder_tree2/2(dout) -> imag_sum/1
  real1/1 -> fir_dbl_tap1/1(a)
  imag1/1 -> fir_dbl_tap1/2(b)
  real_back4/1 -> fir_dbl_tap1/3(c)
  imag_back4/1 -> fir_dbl_tap1/4(d)
  fir_dbl_tap1/1(a_out) -> real_out1/1
  fir_dbl_tap1/2(b_out) -> imag_out1/1
  fir_dbl_tap1/3(c_out) -> real_back_out4/1
  fir_dbl_tap1/4(d_out) -> imag_back_out4/1
  fir_dbl_tap1/5(real) -> adder_tree1/2(din1)
  fir_dbl_tap1/6(imag) -> adder_tree2/2(din1)
  real2/1 -> fir_dbl_tap2/1(a)
  imag2/1 -> fir_dbl_tap2/2(b)
  real_back3/1 -> fir_dbl_tap2/3(c)
  imag_back3/1 -> fir_dbl_tap2/4(d)
  fir_dbl_tap2/1(a_out) -> real_out2/1
  fir_dbl_tap2/2(b_out) -> imag_out2/1
  fir_dbl_tap2/3(c_out) -> real_back_out3/1
  fir_dbl_tap2/4(d_out) -> imag_back_out3/1
  fir_dbl_tap2/5(real) -> adder_tree1/3(din2)
  fir_dbl_tap2/6(imag) -> adder_tree2/3(din2)
  real3/1 -> fir_dbl_tap3/1
  imag3/1 -> fir_dbl_tap3/2
  real_back2/1 -> fir_dbl_tap3/3
  imag_back2/1 -> fir_dbl_tap3/4
  fir_dbl_tap3/1 -> real_out3/1
  fir_dbl_tap3/2 -> imag_out3/1
  fir_dbl_tap3/3 -> real_back_out2/1
  fir_dbl_tap3/4 -> imag_back_out2/1
  fir_dbl_tap3/5 -> adder_tree1/4(din3)
  fir_dbl_tap3/6 -> adder_tree2/4(din3)
  real4/1 -> fir_dbl_tap4/1
  imag4/1 -> fir_dbl_tap4/2
  real_back1/1 -> fir_dbl_tap4/3
  imag_back1/1 -> fir_dbl_tap4/4
  fir_dbl_tap4/1 -> real_out4/1
  fir_dbl_tap4/2 -> imag_out4/1
  fir_dbl_tap4/3 -> real_back_out1/1
  fir_dbl_tap4/4 -> imag_back_out1/1
  fir_dbl_tap4/5 -> adder_tree1/5(din4)
  fir_dbl_tap4/6 -> adder_tree2/5(din4)

== system adc_to_xaui_v2_ddc/dec_fir/imag_sum ==
  sync : Inport  Port=1  LatchInput=off
  din1 : Inport  Port=2  LatchInput=off
  din2 : Inport  Port=3  LatchInput=off
  addr1 : xbsIndex_r3/AddSub  mode=Addition  precision=Full  arith_type=Unsigned  n_bits=8  bin_pt=2  quantization=Truncate  overflow=Wrap  latency=2  explicit_period=off  period=1  use_carryin=off  use_carryout=off  en=off  dbl_ovrd=off  show_param=off  use_core=on  pipeline=on  use_rpm=on  gen_core=off
      settings: xl_area=[0, 0, 0, 0, 0, 0, 0]
  sync_delay : xbsIndex_r3/Delay  latency=2  reg_retiming=off  explicit_period=off  period=1  en=off  accept_only_valid=off  init_zero=on  dbl_ovrd=off  show_param=off
      settings: xl_area=[0, 0, 0, 0, 0, 0, 0]
  sync_out : Outport
  dout : Outport  Port=2
  wires:
  sync/1 -> sync_delay/1
  sync_delay/1 -> sync_out/1
  din1/1 -> addr1/1
  din2/1 -> addr1/2
  addr1/1 -> dout/1

== system adc_to_xaui_v2_ddc/dec_fir/real_sum ==
  sync : Inport  Port=1  LatchInput=off
  din1 : Inport  Port=2  LatchInput=off
  din2 : Inport  Port=3  LatchInput=off
  addr1 : xbsIndex_r3/AddSub  mode=Addition  precision=Full  arith_type=Unsigned  n_bits=8  bin_pt=2  quantization=Truncate  overflow=Wrap  latency=2  explicit_period=off  period=1  use_carryin=off  use_carryout=off  en=off  dbl_ovrd=off  show_param=off  use_core=on  pipeline=on  use_rpm=on  gen_core=off
      settings: xl_area=[0, 0, 0, 0, 0, 0, 0]
  sync_delay : xbsIndex_r3/Delay  latency=2  reg_retiming=off  explicit_period=off  period=1  en=off  accept_only_valid=off  init_zero=on  dbl_ovrd=off  show_param=off
      settings: xl_area=[0, 0, 0, 0, 0, 0, 0]
  sync_out : Outport
  dout : Outport  Port=2
  wires:
  sync/1 -> sync_delay/1
  sync_delay/1 -> sync_out/1
  din1/1 -> addr1/1
  din2/1 -> addr1/2
  addr1/1 -> dout/1

== system adc_to_xaui_v2_ddc/dec_fir/ri_to_c ==
  re : Inport  Port=1  LatchInput=off
  im : Inport  Port=2  LatchInput=off
  Concat : xbsIndex_r3/Concat  num_inputs=2  explicit_period=off  period=1  dbl_ovrd=off
  Reinterpret : xbsIndex_r3/Reinterpret  force_arith_type=on  arith_type=Unsigned  force_bin_pt=on  bin_pt=0  force_valid=on
  Reinterpret1 : xbsIndex_r3/Reinterpret  force_arith_type=on  arith_type=Unsigned  force_bin_pt=on  bin_pt=0  force_valid=on
  c : Outport
  wires:
  Reinterpret/1 -> Concat/1
  Reinterpret1/1 -> Concat/2
  re/1 -> Reinterpret/1
  Concat/1 -> c/1
  im/1 -> Reinterpret1/1

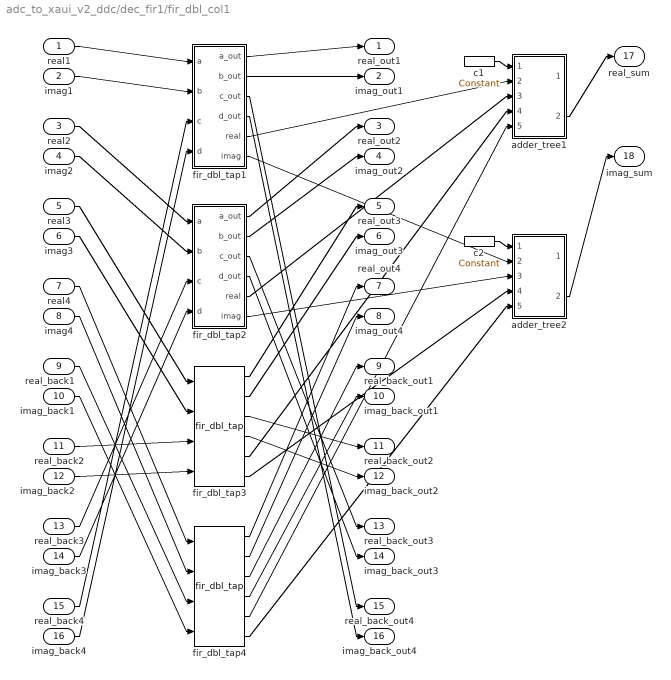
== system adc_to_xaui_v2_ddc/dec_fir1/fir_dbl_col1 ==
  real1 : Inport  Port=1  LatchInput=off
  imag1 : Inport  Port=2  LatchInput=off
  real2 : Inport  Port=3  LatchInput=off
  imag2 : Inport  Port=4  LatchInput=off
  real3 : Inport  Port=5  LatchInput=off
  imag3 : Inport  Port=6  LatchInput=off
  real4 : Inport  Port=7  LatchInput=off
  imag4 : Inport  Port=8  LatchInput=off
  real_back1 : Inport  Port=9  LatchInput=off
  imag_back1 : Inport  Port=10  LatchInput=off
  real_back2 : Inport  Port=11  LatchInput=off
  imag_back2 : Inport  Port=12  LatchInput=off
  real_back3 : Inport  Port=13  LatchInput=off
  imag_back3 : Inport  Port=14  LatchInput=off
  real_back4 : Inport  Port=15  LatchInput=off
  imag_back4 : Inport  Port=16  LatchInput=off
  adder_tree1 : Subsystem  AncestorBlock=casper_library/Misc/adder_tree  mask(adder_tree){n_inputs=4, latency=2}
      mask prompts: n_inputs "Number of Inputs"; latency "Add Latency"
      mask help: Sums all inputs using a tree of adds and delays.
      mask init:
      | adder_tree_init(gcb, ...
      |     'n_inputs', n_inputs, ...
      |     'latency', latency);
      settings: AttributesFormatString=latency 4
      mask Help: eval('xlWeb([getenv(''MLIB_ROOT''), ''\doc\html\sp_adder_tree\sp_adder_tree.html''])')
  adder_tree2 : Subsystem  AncestorBlock=casper_library/Misc/adder_tree  mask(adder_tree){n_inputs=4, latency=2}
      mask prompts: n_inputs "Number of Inputs"; latency "Add Latency"
      mask help: Sums all inputs using a tree of adds and delays.
      mask init:
      | adder_tree_init(gcb, ...
      |     'n_inputs', n_inputs, ...
      |     'latency', latency);
      settings: AttributesFormatString=latency 4
      mask Help: eval('xlWeb([getenv(''MLIB_ROOT''), ''\doc\html\sp_adder_tree\sp_adder_tree.html''])')
  c1 : xbsIndex_r3/Constant  const=1  equ=P=C  arith_type=Unsigned  n_bits=1  bin_pt=0  opselect=C  inp2=PCIN>>17  opr=+  inp1=P  carry=CIN  iostate=0  explicit_period=on  period=1  dbl_ovrd=off
  c2 : xbsIndex_r3/Constant  const=1  equ=P=C  arith_type=Unsigned  n_bits=1  bin_pt=0  opselect=C  inp2=PCIN>>17  opr=+  inp1=P  carry=CIN  iostate=0  explicit_period=on  period=1  dbl_ovrd=off
  fir_dbl_tap1 : Subsystem  AncestorBlock=casper_library/Downconverter/fir_dbl_tap  mask(fir_dbl_tap){factor=-0.02241, add_latency=2, mult_latency=2}
      mask prompts: add_latency "Add latency"; mult_latency "Mult latency"
  fir_dbl_tap2 : Subsystem  AncestorBlock=casper_library/Downconverter/fir_dbl_tap  mask(fir_dbl_tap){factor=-0.04536, add_latency=2, mult_latency=2}
      mask prompts: add_latency "Add latency"; mult_latency "Mult latency"
  fir_dbl_tap3 : casper_library/Downconverter/fir_dbl_tap  factor=-0.03852  add_latency=2  mult_latency=2
      link override Constant: equ=P=C
  fir_dbl_tap4 : casper_library/Downconverter/fir_dbl_tap  factor=-0.01449  add_latency=2  mult_latency=2
      link override Constant: equ=P=C
  real_out1 : Outport
  imag_out1 : Outport  Port=2
  real_out2 : Outport  Port=3
  imag_out2 : Outport  Port=4
  real_out3 : Outport  Port=5
  imag_out3 : Outport  Port=6
  real_out4 : Outport  Port=7
  imag_out4 : Outport  Port=8
  real_back_out1 : Outport  Port=9
  imag_back_out1 : Outport  Port=10
  real_back_out2 : Outport  Port=11
  imag_back_out2 : Outport  Port=12
  real_back_out3 : Outport  Port=13
  imag_back_out3 : Outport  Port=14
  real_back_out4 : Outport  Port=15
  imag_back_out4 : Outport  Port=16
  real_sum : Outport  Port=17
  imag_sum : Outport  Port=18
  wires:
  c1/1 -> adder_tree1/1(sync)
  c2/1 -> adder_tree2/1(sync)
  adder_tree1/2(dout) -> real_sum/1
  adder_tree2/2(dout) -> imag_sum/1
  real1/1 -> fir_dbl_tap1/1(a)
  imag1/1 -> fir_dbl_tap1/2(b)
  real_back4/1 -> fir_dbl_tap1/3(c)
  imag_back4/1 -> fir_dbl_tap1/4(d)
  fir_dbl_tap1/1(a_out) -> real_out1/1
  fir_dbl_tap1/2(b_out) -> imag_out1/1
  fir_dbl_tap1/3(c_out) -> real_back_out4/1
  fir_dbl_tap1/4(d_out) -> imag_back_out4/1
  fir_dbl_tap1/5(real) -> adder_tree1/2(din1)
  fir_dbl_tap1/6(imag) -> adder_tree2/2(din1)
  real2/1 -> fir_dbl_tap2/1(a)
  imag2/1 -> fir_dbl_tap2/2(b)
  real_back3/1 -> fir_dbl_tap2/3(c)
  imag_back3/1 -> fir_dbl_tap2/4(d)
  fir_dbl_tap2/1(a_out) -> real_out2/1
  fir_dbl_tap2/2(b_out) -> imag_out2/1
  fir_dbl_tap2/3(c_out) -> real_back_out3/1
  fir_dbl_tap2/4(d_out) -> imag_back_out3/1
  fir_dbl_tap2/5(real) -> adder_tree1/3(din2)
  fir_dbl_tap2/6(imag) -> adder_tree2/3(din2)
  real3/1 -> fir_dbl_tap3/1
  imag3/1 -> fir_dbl_tap3/2
  real_back2/1 -> fir_dbl_tap3/3
  imag_back2/1 -> fir_dbl_tap3/4
  fir_dbl_tap3/1 -> real_out3/1
  fir_dbl_tap3/2 -> imag_out3/1
  fir_dbl_tap3/3 -> real_back_out2/1
  fir_dbl_tap3/4 -> imag_back_out2/1
  fir_dbl_tap3/5 -> adder_tree1/4(din3)
  fir_dbl_tap3/6 -> adder_tree2/4(din3)
  real4/1 -> fir_dbl_tap4/1
  imag4/1 -> fir_dbl_tap4/2
  real_back1/1 -> fir_dbl_tap4/3
  imag_back1/1 -> fir_dbl_tap4/4
  fir_dbl_tap4/1 -> real_out4/1
  fir_dbl_tap4/2 -> imag_out4/1
  fir_dbl_tap4/3 -> real_back_out1/1
  fir_dbl_tap4/4 -> imag_back_out1/1
  fir_dbl_tap4/5 -> adder_tree1/5(din4)
  fir_dbl_tap4/6 -> adder_tree2/5(din4)
